simulink model "Receive1"  (R2021a)
settings: Solver=VariableStepAuto  StartTime=0.0  StopTime=20000  RelTol=1e-3
values from neighbouring files (symbols this model uses):
  n_overlapped_channel = 2 * 1024    (= 2048)    [receive1_script.m]
  parallel_factor = 4    [receive1_script.m]
libraries: xbsIndex_r4 x522, xrbsSSR_Library x15, dspsrcs4 x12
(part 2 of 4)

== system Receive1/beat_dphi2 ==
  w_addr : Inport
  w_data : Inport  Port=2
  we : Inport  Port=3
  tvalid_in : Inport  Port=4
  AddSub : xbsIndex_r4/AddSub  mode=Addition  use_carryin=off  use_carryout=off  en=off  latency=2  precision=User Defined  arith_type=Unsigned  n_bits=16  bin_pt=0  quantization=Truncate  overflow=Wrap  use_behavioral_HDL=off  hw_selection=Fabric  pipelined=off  dbl_ovrd=off  block_type=addsub
  Constant3 : xbsIndex_r4/Constant  const=0  gui_display_data_type=Boolean  arith_type=Boolean  n_bits=16  bin_pt=14  preci_type=Single  exp_width=8  frac_width=24  explicit_period=on  period=1  equ=P=C  opselect=C  inp2=PCIN>>17  opr=+  inp1=P  carry=CIN  dbl_ovrd=off  block_type=constant
  Constant5 : xbsIndex_r4/Constant  const=0  gui_display_data_type=Fixed-point  arith_type=Unsigned  n_bits=16  bin_pt=0  preci_type=Single  exp_width=8  frac_width=24  explicit_period=on  period=1  equ=P=C  opselect=C  inp2=PCIN>>17  opr=+  inp1=P  carry=CIN  dbl_ovrd=off  block_type=constant
  Constant6 : xbsIndex_r4/Constant  const=1  gui_display_data_type=Boolean  arith_type=Boolean  n_bits=16  bin_pt=14  preci_type=Single  exp_width=8  frac_width=24  explicit_period=on  period=1  equ=P=C  opselect=C  inp2=PCIN>>17  opr=+  inp1=P  carry=CIN  dbl_ovrd=off  block_type=constant
  Constant8 : xbsIndex_r4/Constant  const=0  gui_display_data_type=Fixed-point  arith_type=Unsigned  n_bits=16  bin_pt=0  preci_type=Single  exp_width=8  frac_width=24  explicit_period=on  period=1  equ=P=C  opselect=C  inp2=PCIN>>17  opr=+  inp1=P  carry=CIN  dbl_ovrd=off  block_type=constant
  Convert2 : xbsIndex_r4/Convert  gui_display_data_type=Fixed-point  arith_type="Signed  (2's comp)"  n_bits=18  bin_pt=15  float_type=Single  exp_bits=8  fraction_bits=24  quantization=Truncate  overflow=Wrap  en=off  latency=0  pipeline=off  dbl_ovrd=off  block_type=convert
  Counter2 : xbsIndex_r4/Counter  cnt_type=Free Running  cnt_to=Inf  operation=Up  start_count=0  cnt_by_val=1  arith_type=Unsigned  n_bits=9  bin_pt=0  load_pin=off  rst=on  en=on  explicit_period=on  period=1  use_behavioral_HDL=off  implementation=Fabric  dbl_ovrd=off  block_type=counter
  Delay{1,16,37..38} (4 alike) : xbsIndex_r4/Delay  rst=off  infoeditControl=Selection of Reset will increase slice count due to use of real FFs and instead of SRLs  en=off  latency=1  reg_retiming=off  dbl_ovrd=off  block_type=delay
  Delay17 : xbsIndex_r4/Delay  rst=off  infoeditControl=Selection of Reset will increase slice count due to use of real FFs and instead of SRLs  en=off  latency=n_overlapped_channel/parallel_factor-2-1-1  reg_retiming=off  dbl_ovrd=off  block_type=delay
  Dual Port RAM : xbsIndex_r4/Dual Port RAM  depth=n_overlapped_channel/parallel_factor  initVector=beat_dphi_uint16_2  distributed_mem=Block RAM  init_a=0  init_b=0  rst_a=off  rst_b=off  en_a=off  en_b=off  latency=1  write_mode_A=Read Before Write  write_mode_B=Read Before Write  optimize=Area  dbl_ovrd=off  simulation_type=fast_sim  block_type=dpram
  FIFO4 : xbsIndex_r4/FIFO  mem_type=Block RAM  performance_options=Standard_FIFO  embedded_registers=off  depth=1K  percent_nbits=1  rst=off  rst_latency=2  en=off  use_dcount=off  use_percent_full_port=off  use_almost_empty=off  almost_empty_thresh=2  use_almost_full=off  use_rd_rst_busy=off  use_wr_rst_busy=off  almost_full_thresh=14  explicit_period=off  dbl_ovrd=off  simulation_type=fast_sim  block_type=fifo
  Mux1 : xbsIndex_r4/Mux  inputs=2  en=off  latency=1  precision=User Defined  arith_type=Unsigned  n_bits=16  bin_pt=0  quantization=Truncate  overflow=Flag as error  dbl_ovrd=off  block_type=mux
  Mux2 : xbsIndex_r4/Mux  inputs=2  en=off  latency=1  precision=User Defined  arith_type=Unsigned  n_bits=16  bin_pt=0  quantization=Truncate  overflow=Flag as error  dbl_ovrd=off  block_type=mux
  Reinterpret2 : xbsIndex_r4/Reinterpret  force_arith_type=on  arith_type="Signed  (2's comp)"  force_bin_pt=on  bin_pt=15  block_type=reinterpret
  Terminator : Terminator
  Terminator11 : Terminator
  Terminator9 : Terminator
  rst_det : Subsystem
  beat_dphi : Outport
  wires:
  FIFO4/1 -> Mux1/3
  Reinterpret2/1 -> Convert2/1
  Delay17/1 -> FIFO4/3
  Delay38/1 -> Dual Port RAM/4
  Delay37/1 -> Dual Port RAM/5
  Delay16/1 -> Dual Port RAM/6
  Constant3/1 -> Dual Port RAM/3
  AddSub/1 -> FIFO4/1
  Constant6/1 -> FIFO4/2, Delay17/1
  FIFO4/3 -> Terminator11/1
  Constant8/1 -> Dual Port RAM/2
  FIFO4/2 -> Terminator9/1
  Dual Port RAM/2 -> Terminator/1
  Counter2/1 -> Dual Port RAM/1
  Constant5/1 -> Mux2/2, Mux1/2
  Mux2/1 -> AddSub/1
  w_data/1 -> Delay37/1
  Dual Port RAM/1 -> Mux2/3
  Convert2/1 -> beat_dphi/1
  w_addr/1 -> Delay38/1
  we/1 -> Delay16/1
  tvalid_in/1 -> rst_det/1(in), Delay1/1, Counter2/2
  rst_det/1(out) -> Counter2/1
  Delay1/1 -> Mux1/1, Mux2/1
  Mux1/1 -> Reinterpret2/1, AddSub/2

== system Receive1/beat_dphi3 ==
  w_addr : Inport
  w_data : Inport  Port=2
  we : Inport  Port=3
  tvalid_in : Inport  Port=4
  AddSub : xbsIndex_r4/AddSub  mode=Addition  use_carryin=off  use_carryout=off  en=off  latency=2  precision=User Defined  arith_type=Unsigned  n_bits=16  bin_pt=0  quantization=Truncate  overflow=Wrap  use_behavioral_HDL=off  hw_selection=Fabric  pipelined=off  dbl_ovrd=off  block_type=addsub
  Constant3 : xbsIndex_r4/Constant  const=0  gui_display_data_type=Boolean  arith_type=Boolean  n_bits=16  bin_pt=14  preci_type=Single  exp_width=8  frac_width=24  explicit_period=on  period=1  equ=P=C  opselect=C  inp2=PCIN>>17  opr=+  inp1=P  carry=CIN  dbl_ovrd=off  block_type=constant
  Constant5 : xbsIndex_r4/Constant  const=0  gui_display_data_type=Fixed-point  arith_type=Unsigned  n_bits=16  bin_pt=0  preci_type=Single  exp_width=8  frac_width=24  explicit_period=on  period=1  equ=P=C  opselect=C  inp2=PCIN>>17  opr=+  inp1=P  carry=CIN  dbl_ovrd=off  block_type=constant
  Constant6 : xbsIndex_r4/Constant  const=1  gui_display_data_type=Boolean  arith_type=Boolean  n_bits=16  bin_pt=14  preci_type=Single  exp_width=8  frac_width=24  explicit_period=on  period=1  equ=P=C  opselect=C  inp2=PCIN>>17  opr=+  inp1=P  carry=CIN  dbl_ovrd=off  block_type=constant
  Constant8 : xbsIndex_r4/Constant  const=0  gui_display_data_type=Fixed-point  arith_type=Unsigned  n_bits=16  bin_pt=0  preci_type=Single  exp_width=8  frac_width=24  explicit_period=on  period=1  equ=P=C  opselect=C  inp2=PCIN>>17  opr=+  inp1=P  carry=CIN  dbl_ovrd=off  block_type=constant
  Convert2 : xbsIndex_r4/Convert  gui_display_data_type=Fixed-point  arith_type="Signed  (2's comp)"  n_bits=18  bin_pt=15  float_type=Single  exp_bits=8  fraction_bits=24  quantization=Truncate  overflow=Wrap  en=off  latency=0  pipeline=off  dbl_ovrd=off  block_type=convert
  Counter2 : xbsIndex_r4/Counter  cnt_type=Free Running  cnt_to=Inf  operation=Up  start_count=0  cnt_by_val=1  arith_type=Unsigned  n_bits=9  bin_pt=0  load_pin=off  rst=on  en=on  explicit_period=on  period=1  use_behavioral_HDL=off  implementation=Fabric  dbl_ovrd=off  block_type=counter
  Delay{1,16,37..38} (4 alike) : xbsIndex_r4/Delay  rst=off  infoeditControl=Selection of Reset will increase slice count due to use of real FFs and instead of SRLs  en=off  latency=1  reg_retiming=off  dbl_ovrd=off  block_type=delay
  Delay17 : xbsIndex_r4/Delay  rst=off  infoeditControl=Selection of Reset will increase slice count due to use of real FFs and instead of SRLs  en=off  latency=n_overlapped_channel/parallel_factor-2-1-1  reg_retiming=off  dbl_ovrd=off  block_type=delay
  Dual Port RAM : xbsIndex_r4/Dual Port RAM  depth=n_overlapped_channel/parallel_factor  initVector=beat_dphi_uint16_3  distributed_mem=Block RAM  init_a=0  init_b=0  rst_a=off  rst_b=off  en_a=off  en_b=off  latency=1  write_mode_A=Read Before Write  write_mode_B=Read Before Write  optimize=Area  dbl_ovrd=off  simulation_type=fast_sim  block_type=dpram
  FIFO4 : xbsIndex_r4/FIFO  mem_type=Block RAM  performance_options=Standard_FIFO  embedded_registers=off  depth=1K  percent_nbits=1  rst=off  rst_latency=2  en=off  use_dcount=off  use_percent_full_port=off  use_almost_empty=off  almost_empty_thresh=2  use_almost_full=off  use_rd_rst_busy=off  use_wr_rst_busy=off  almost_full_thresh=14  explicit_period=off  dbl_ovrd=off  simulation_type=fast_sim  block_type=fifo
  Mux1 : xbsIndex_r4/Mux  inputs=2  en=off  latency=1  precision=User Defined  arith_type=Unsigned  n_bits=16  bin_pt=0  quantization=Truncate  overflow=Flag as error  dbl_ovrd=off  block_type=mux
  Mux2 : xbsIndex_r4/Mux  inputs=2  en=off  latency=1  precision=User Defined  arith_type=Unsigned  n_bits=16  bin_pt=0  quantization=Truncate  overflow=Flag as error  dbl_ovrd=off  block_type=mux
  Reinterpret2 : xbsIndex_r4/Reinterpret  force_arith_type=on  arith_type="Signed  (2's comp)"  force_bin_pt=on  bin_pt=15  block_type=reinterpret
  Terminator : Terminator
  Terminator11 : Terminator
  Terminator9 : Terminator
  rst_det : Subsystem
  beat_dphi : Outport
  wires:
  FIFO4/1 -> Mux1/3
  Reinterpret2/1 -> Convert2/1
  Delay17/1 -> FIFO4/3
  Delay38/1 -> Dual Port RAM/4
  Delay37/1 -> Dual Port RAM/5
  Delay16/1 -> Dual Port RAM/6
  Constant3/1 -> Dual Port RAM/3
  AddSub/1 -> FIFO4/1
  Constant6/1 -> FIFO4/2, Delay17/1
  FIFO4/3 -> Terminator11/1
  Constant8/1 -> Dual Port RAM/2
  FIFO4/2 -> Terminator9/1
  Dual Port RAM/2 -> Terminator/1
  Counter2/1 -> Dual Port RAM/1
  Constant5/1 -> Mux2/2, Mux1/2
  Mux2/1 -> AddSub/1
  w_data/1 -> Delay37/1
  Dual Port RAM/1 -> Mux2/3
  Convert2/1 -> beat_dphi/1
  w_addr/1 -> Delay38/1
  we/1 -> Delay16/1
  tvalid_in/1 -> rst_det/1(in), Delay1/1, Counter2/2
  rst_det/1(out) -> Counter2/1
  Delay1/1 -> Mux1/1, Mux2/1
  Mux1/1 -> Reinterpret2/1, AddSub/2

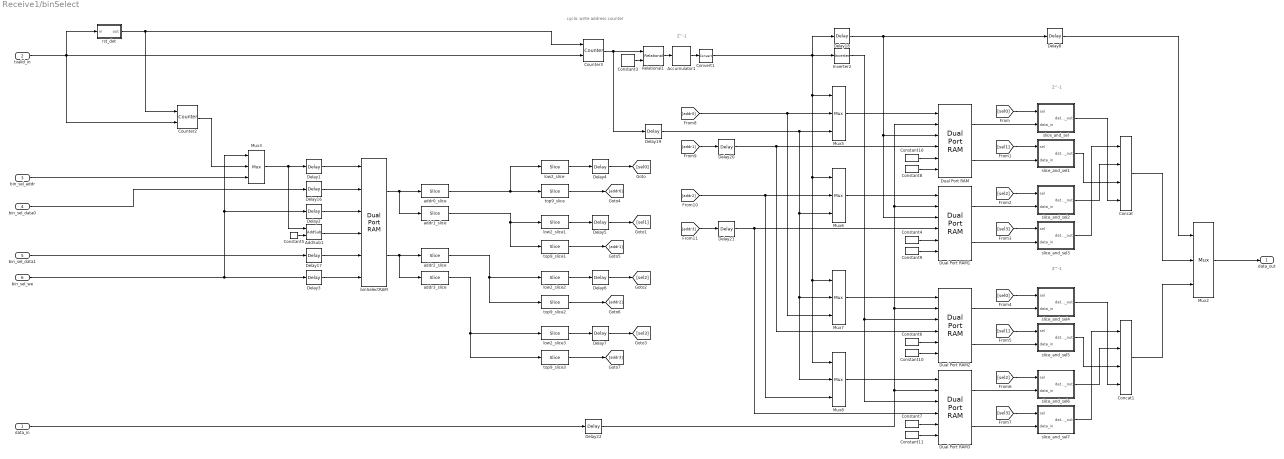
== system Receive1/binSelect ==
  note: Z^-1
  note: Z^-1
  note: Z^-1
  note: cyclic write address counter
  data_in : Inport
  tvalid_in : Inport  Port=2
  bin_sel_addr : Inport  Port=3
  bin_sel_data0 : Inport  Port=4
  bin_sel_data1 : Inport  Port=5
  bin_sel_we : Inport  Port=6
  Accumulator1 : xbsIndex_r4/Accumulator  operation=Add  n_bits=1  overflow=Wrap  scale=1  rst=off  hasbypass=off  infoeditControl=reset for floating point data type must be asserted for a minimum of 2 cycles  en=off  latency=1  msb_inp=100  msb=100  lsb=-100  use_behavioral_HDL=on  implementation=Fabric  dbl_ovrd=off  block_type=accum
  AddSub1 : xbsIndex_r4/AddSub  mode=Addition  use_carryin=off  use_carryout=off  en=off  latency=1  precision=User Defined  arith_type=Unsigned  n_bits=10  bin_pt=0  quantization=Truncate  overflow=Wrap  use_behavioral_HDL=on  hw_selection=Fabric  pipelined=on  dbl_ovrd=off  block_type=addsub
      settings: SourceProductName=Attempt to write the readonly database /home/ugrad/.matlab/R2018a/slblocks_master.db. (attempt to write a readonly database)
  Concat : xbsIndex_r4/Concat  num_inputs=4  dbl_ovrd=off  block_type=concat
  Concat1 : xbsIndex_r4/Concat  num_inputs=4  dbl_ovrd=off  block_type=concat
  Constant{8..11} (4 alike) : xbsIndex_r4/Constant  const=0  gui_display_data_type=Boolean  arith_type=Boolean  n_bits=1  bin_pt=0  preci_type=Single  exp_width=8  frac_width=24  explicit_period=on  period=1  equ=P=C  opselect=C  inp2=PCIN>>17  opr=+  inp1=P  carry=CIN  dbl_ovrd=off  block_type=constant
      settings: SourceProductName=Attempt to write the readonly database /home/ugrad/.matlab/R2018a/slblocks_master.db. (attempt to write a readonly database)
  Constant{4,6..7,16} (4 alike) : xbsIndex_r4/Constant  const=0  gui_display_data_type=Fixed-point  arith_type=Unsigned  n_bits=216  bin_pt=0  preci_type=Single  exp_width=8  frac_width=24  explicit_period=on  period=1  equ=P=C  opselect=C  inp2=PCIN>>17  opr=+  inp1=P  carry=CIN  dbl_ovrd=off  block_type=constant
      settings: SourceProductName=Attempt to write the readonly database /home/ugrad/.matlab/R2018a/slblocks_master.db. (attempt to write a readonly database)
  Constant3 : xbsIndex_r4/Constant  const=n_overlapped_channel/parallel_factor - 1  gui_display_data_type=Fixed-point  arith_type=Unsigned  n_bits=9  bin_pt=0  preci_type=Single  exp_width=8  frac_width=24  explicit_period=on  period=1  equ=P=C  opselect=C  inp2=PCIN>>17  opr=+  inp1=P  carry=CIN  dbl_ovrd=off  block_type=constant
  Constant5 : xbsIndex_r4/Constant  const=1  gui_display_data_type=Fixed-point  arith_type=Unsigned  n_bits=10  bin_pt=0  preci_type=Single  exp_width=8  frac_width=24  explicit_period=on  period=1  equ=P=C  opselect=C  inp2=PCIN>>17  opr=+  inp1=P  carry=CIN  dbl_ovrd=off  block_type=constant
      settings: SourceProductName=Attempt to write the readonly database /home/ugrad/.matlab/R2018a/slblocks_master.db. (attempt to write a readonly database)
  Convert1 : xbsIndex_r4/Convert  gui_display_data_type=Boolean  arith_type=Boolean  n_bits=16  bin_pt=14  float_type=Single  exp_bits=8  fraction_bits=24  quantization=Truncate  overflow=Wrap  en=off  latency=1  pipeline=off  dbl_ovrd=off  block_type=convert
  Counter2 : xbsIndex_r4/Counter  cnt_type=Free Running  cnt_to=Inf  operation=Up  start_count=0  cnt_by_val=2  arith_type=Unsigned  n_bits=10  bin_pt=0  load_pin=off  rst=on  en=on  explicit_period=on  period=1  use_behavioral_HDL=off  implementation=Fabric  dbl_ovrd=off  block_type=counter
  Counter3 : xbsIndex_r4/Counter  cnt_type=Free Running  cnt_to=Inf  operation=Up  start_count=0  cnt_by_val=1  arith_type=Unsigned  n_bits=9  bin_pt=0  load_pin=off  rst=on  en=on  explicit_period=on  period=1  use_behavioral_HDL=off  implementation=Fabric  dbl_ovrd=off  block_type=counter
  Delay{1,18,20..21} (4 alike) : xbsIndex_r4/Delay  rst=off  infoeditControl=Selection of Reset will increase slice count due to use of real FFs and instead of SRLs  en=off  latency=1  reg_retiming=off  dbl_ovrd=off  block_type=delay
  Delay{2..8,16..17} (9 alike) : xbsIndex_r4/Delay  rst=off  infoeditControl=Selection of Reset will increase slice count due to use of real FFs and instead of SRLs  en=off  latency=2  reg_retiming=off  dbl_ovrd=off  block_type=delay
  Delay19 : xbsIndex_r4/Delay  rst=off  infoeditControl=Selection of Reset will increase slice count due to use of real FFs and instead of SRLs  en=off  latency=3  reg_retiming=off  dbl_ovrd=off  block_type=delay
  Delay22 : xbsIndex_r4/Delay  rst=off  infoeditControl=Selection of Reset will increase slice count due to use of real FFs and instead of SRLs  en=off  latency=4  reg_retiming=off  dbl_ovrd=off  block_type=delay
  Dual Port RAM{,1..3} (4 alike) : xbsIndex_r4/Dual Port RAM  depth=n_overlapped_channel/parallel_factor  initVector=0  distributed_mem=Block RAM  init_a=0  init_b=0  rst_a=off  rst_b=off  en_a=off  en_b=off  latency=1  write_mode_A=Read Before Write  write_mode_B=Read Before Write  optimize=Area  dbl_ovrd=off  simulation_type=fast_sim  block_type=dpram
  Inverter2 : xbsIndex_r4/Inverter  en=off  latency=1  dbl_ovrd=off  block_type=inv
  Mux{2..3,5..8} (6 alike) : xbsIndex_r4/Mux  inputs=2  en=off  latency=1  precision=Full  arith_type=Unsigned  n_bits=16  bin_pt=14  quantization=Truncate  overflow=Wrap  dbl_ovrd=off  block_type=mux
  Relational1 : xbsIndex_r4/Relational  mode=a=b  op_type=Ufix  en=off  latency=1  dbl_ovrd=off  block_type=relational
  addr0_slice : xbsIndex_r4/Slice  nbits=11  boolean_output=off  mode=Lower Bit Location + Width  bit1=0  base1=MSB of Input  bit0=0  base0=LSB of Input  dbl_ovrd=off  block_type=slice
  addr1_slice : xbsIndex_r4/Slice  nbits=11  boolean_output=off  mode=Lower Bit Location + Width  bit1=0  base1=MSB of Input  bit0=11  base0=LSB of Input  dbl_ovrd=off  block_type=slice
  addr2_slice : xbsIndex_r4/Slice  nbits=11  boolean_output=off  mode=Lower Bit Location + Width  bit1=0  base1=MSB of Input  bit0=0  base0=LSB of Input  dbl_ovrd=off  block_type=slice
  addr3_slice : xbsIndex_r4/Slice  nbits=11  boolean_output=off  mode=Lower Bit Location + Width  bit1=0  base1=MSB of Input  bit0=11  base0=LSB of Input  dbl_ovrd=off  block_type=slice
  binSelectRAM : xbsIndex_r4/Dual Port RAM  depth=2*n_overlapped_channel/parallel_factor  initVector=bin_map  distributed_mem=Block RAM  init_a=0  init_b=0  rst_a=off  rst_b=off  en_a=off  en_b=off  latency=1  write_mode_A=Read Before Write  write_mode_B=Read Before Write  optimize=Area  dbl_ovrd=off  simulation_type=fast_sim  block_type=dpram
  low2_slice{,1..3} (4 alike) : xbsIndex_r4/Slice  nbits=2  boolean_output=off  mode=Lower Bit Location + Width  bit1=0  base1=MSB of Input  bit0=0  base0=LSB of Input  dbl_ovrd=off  block_type=slice
  rst_det : Subsystem
  slice_and_sel : Subsystem
  slice_and_sel1 : Subsystem
  slice_and_sel2 : Subsystem
  slice_and_sel3 : Subsystem
  slice_and_sel4 : Subsystem
  slice_and_sel5 : Subsystem
  slice_and_sel6 : Subsystem
  slice_and_sel7 : Subsystem
  top9_slice{,1..3} (4 alike) : xbsIndex_r4/Slice  nbits=9  boolean_output=off  mode=Lower Bit Location + Width  bit1=0  base1=MSB of Input  bit0=2  base0=LSB of Input  dbl_ovrd=off  block_type=slice
  data_out : Outport
  wires:
  [sel0] -> slice_and_sel/1(sel)
  Dual Port RAM/1 -> slice_and_sel/2(data_in)
  Dual Port RAM/2 -> slice_and_sel1/2(data_in)
  Dual Port RAM1/1 -> slice_and_sel2/2(data_in)
  Dual Port RAM1/2 -> slice_and_sel3/2(data_in)
  [sel1] -> slice_and_sel1/1(sel)
  [sel2] -> slice_and_sel2/1(sel)
  [sel3] -> slice_and_sel3/1(sel)
  slice_and_sel/1(data_out) -> Concat/4
  slice_and_sel1/1(data_out) -> Concat/3
  slice_and_sel2/1(data_out) -> Concat/2
  slice_and_sel3/1(data_out) -> Concat/1
  Dual Port RAM2/2 -> slice_and_sel5/2(data_in)
  slice_and_sel5/1(data_out) -> Concat1/3
  [sel0] -> slice_and_sel4/1(sel)
  Dual Port RAM2/1 -> slice_and_sel4/2(data_in)
  slice_and_sel7/1(data_out) -> Concat1/1
  [sel3] -> slice_and_sel7/1(sel)
  Dual Port RAM3/2 -> slice_and_sel7/2(data_in)
  [sel2] -> slice_and_sel6/1(sel)
  Dual Port RAM3/1 -> slice_and_sel6/2(data_in)
  [sel1] -> slice_and_sel5/1(sel)
  slice_and_sel4/1(data_out) -> Concat1/4
  slice_and_sel6/1(data_out) -> Concat1/2
  Concat/1 -> Mux2/2
  Concat1/1 -> Mux2/3
  Mux2/1 -> data_out/1
  Constant5/1 -> AddSub1/2
  AddSub1/1 -> binSelectRAM/4
  Delay1/1 -> binSelectRAM/1
  Mux3/1 -> Delay1/1, AddSub1/1
  Counter2/1 -> Mux3/2
  bin_sel_we/1 -> Delay2/1, Mux3/1, Delay3/1
  bin_sel_addr/1 -> Mux3/3
  Delay3/1 -> binSelectRAM/6
  Delay2/1 -> binSelectRAM/3
  Delay16/1 -> binSelectRAM/2
  Delay17/1 -> binSelectRAM/5
  bin_sel_data0/1 -> Delay16/1
  bin_sel_data1/1 -> Delay17/1
  binSelectRAM/1 -> addr0_slice/1, addr1_slice/1
  binSelectRAM/2 -> addr2_slice/1, addr3_slice/1
  addr0_slice/1 -> top9_slice/1, low2_slice/1
  addr1_slice/1 -> top9_slice1/1, low2_slice1/1
  addr2_slice/1 -> top9_slice2/1, low2_slice2/1
  addr3_slice/1 -> top9_slice3/1, low2_slice3/1
  top9_slice3/1 -> [addr3]
  top9_slice/1 -> [addr0]
  top9_slice1/1 -> [addr1]
  top9_slice2/1 -> [addr2]
  Mux5/1 -> Dual Port RAM/1
  Mux6/1 -> Dual Port RAM1/1
  Mux7/1 -> Dual Port RAM2/1
  Mux8/1 -> Dual Port RAM3/1
  Constant3/1 -> Relational1/2
  Accumulator1/1 -> Convert1/1
  Counter3/1 -> Delay19/1, Relational1/1
  Relational1/1 -> Accumulator1/1
  Constant16/1 -> Dual Port RAM/5
  Constant4/1 -> Dual Port RAM1/5
  Constant6/1 -> Dual Port RAM2/5
  Constant7/1 -> Dual Port RAM3/5
  Constant8/1 -> Dual Port RAM/6
  Constant9/1 -> Dual Port RAM1/6
  Constant10/1 -> Dual Port RAM2/6
  Constant11/1 -> Dual Port RAM3/6
  Convert1/1 -> Mux5/1, Mux8/1, Mux7/1, Mux6/1, Delay18/1, Inverter2/1
  Delay19/1 -> Mux8/2, Mux7/2, Mux6/3, Mux5/3
  Inverter2/1 -> Dual Port RAM2/3, Dual Port RAM3/3
  Delay18/1 -> Dual Port RAM1/3, Dual Port RAM/3, Delay8/1
  [addr0] -> Mux5/2, Mux7/3
  [addr1] -> Delay20/1
  [addr2] -> Mux6/2, Mux8/3
  [addr3] -> Delay21/1
  Delay20/1 -> Dual Port RAM/4, Dual Port RAM2/4
  Delay21/1 -> Dual Port RAM1/4, Dual Port RAM3/4
  data_in/1 -> Delay22/1
  Delay22/1 -> Dual Port RAM/2, Dual Port RAM1/2, Dual Port RAM2/2, Dual Port RAM3/2
  tvalid_in/1 -> Counter3/2, Counter2/2, rst_det/1(in)
  rst_det/1(out) -> Counter2/1, Counter3/1
  low2_slice/1 -> Delay4/1
  Delay4/1 -> [sel0]
  Delay5/1 -> [sel1]
  low2_slice1/1 -> Delay5/1
  Delay6/1 -> [sel2]
  low2_slice2/1 -> Delay6/1
  Delay7/1 -> [sel3]
  low2_slice3/1 -> Delay7/1
  Delay8/1 -> Mux2/1

== system Receive1/delayCounter ==
  note: Counter that is enabled after the first rising edge1, and disabled after the first rising edge2. Need to calibrate the initial value of counter before getting desired delay value.
  edge1 : Inport
  edge2 : Inport  Port=2
  Counter1 : xbsIndex_r4/Counter  cnt_type=Free Running  cnt_to=Inf  operation=Up  start_count=0  cnt_by_val=1  arith_type=Unsigned  n_bits=12  bin_pt=0  load_pin=off  rst=off  en=on  explicit_period=on  period=1  use_behavioral_HDL=off  implementation=DSP48  dbl_ovrd=off  block_type=counter
  Logical : xbsIndex_r4/Logical  logical_function=XOR  inputs=2  en=off  latency=1  precision=User Defined  arith_type=Boolean  n_bits=1  bin_pt=0  align_bp=on  dbl_ovrd=off  block_type=logical
  Register1 : xbsIndex_r4/Register  init=0  rst=off  en=on  dbl_ovrd=off  block_type=register
  Register2 : xbsIndex_r4/Register  init=0  rst=off  en=on  dbl_ovrd=off  block_type=register
  const1 : xbsIndex_r4/Constant  const=1  gui_display_data_type=Boolean  arith_type=Boolean  n_bits=18  bin_pt=16  preci_type=Single  exp_width=8  frac_width=24  explicit_period=on  period=1  equ=P=C  opselect=C  inp2=PCIN>>17  opr=+  inp1=P  carry=CIN  dbl_ovrd=off  block_type=constant
  delay : Outport
  wires:
  Counter1/1 -> delay/1
  Register2/1 -> Logical/2
  Logical/1 -> Counter1/1
  const1/1 -> Register1/1, Register2/1
  Register1/1 -> Logical/1
  edge2/1 -> Register2/2
  edge1/1 -> Register1/2

== system Receive1/delayCounter1 ==
  note: Counter that is enabled after the first rising edge1, and disabled after the first rising edge2. Need to calibrate the initial value of counter before getting desired delay value.
  edge1 : Inport
  edge2 : Inport  Port=2
  Counter1 : xbsIndex_r4/Counter  cnt_type=Free Running  cnt_to=Inf  operation=Up  start_count=0  cnt_by_val=1  arith_type=Unsigned  n_bits=12  bin_pt=0  load_pin=off  rst=off  en=on  explicit_period=on  period=1  use_behavioral_HDL=off  implementation=DSP48  dbl_ovrd=off  block_type=counter
  Logical : xbsIndex_r4/Logical  logical_function=XOR  inputs=2  en=off  latency=1  precision=User Defined  arith_type=Boolean  n_bits=1  bin_pt=0  align_bp=on  dbl_ovrd=off  block_type=logical
  Register1 : xbsIndex_r4/Register  init=0  rst=off  en=on  dbl_ovrd=off  block_type=register
  Register2 : xbsIndex_r4/Register  init=0  rst=off  en=on  dbl_ovrd=off  block_type=register
  const1 : xbsIndex_r4/Constant  const=1  gui_display_data_type=Boolean  arith_type=Boolean  n_bits=18  bin_pt=16  preci_type=Single  exp_width=8  frac_width=24  explicit_period=on  period=1  equ=P=C  opselect=C  inp2=PCIN>>17  opr=+  inp1=P  carry=CIN  dbl_ovrd=off  block_type=constant
  delay : Outport
  wires:
  Counter1/1 -> delay/1
  Register2/1 -> Logical/2
  Logical/1 -> Counter1/1
  const1/1 -> Register1/1, Register2/1
  Register1/1 -> Logical/1
  edge2/1 -> Register2/2
  edge1/1 -> Register1/2

== system Receive1/rst_det ==
  in : Inport
  Inverter : xbsIndex_r4/Inverter  en=off  latency=1  dbl_ovrd=off  block_type=inv
  Logical : xbsIndex_r4/Logical  logical_function=AND  inputs=2  en=off  latency=1  precision=User Defined  arith_type=Boolean  n_bits=1  bin_pt=0  align_bp=on  dbl_ovrd=off  block_type=logical
  Logical1 : xbsIndex_r4/Logical  logical_function=XOR  inputs=2  en=off  latency=1  precision=User Defined  arith_type=Boolean  n_bits=1  bin_pt=0  align_bp=on  dbl_ovrd=off  block_type=logical
  Register : xbsIndex_r4/Register  init=0  rst=off  en=off  dbl_ovrd=off  block_type=register
  out : Outport
  wires:
  Register/1 -> Logical1/2, Logical/2
  Inverter/1 -> Logical1/1, Register/1
  Logical1/1 -> Logical/1
  in/1 -> Inverter/1
  Logical/1 -> out/1

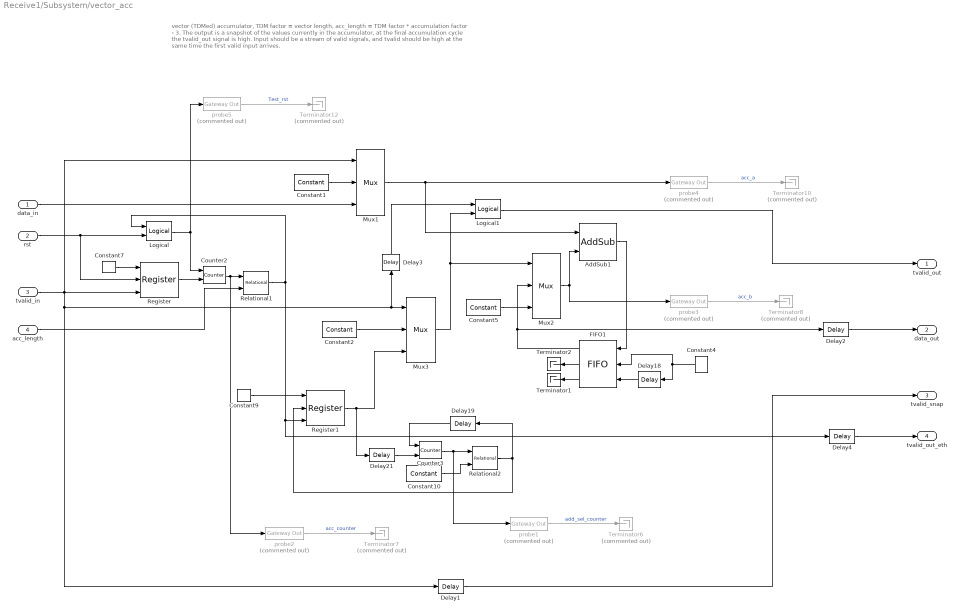
== system Receive1/Subsystem/vector_acc ==
  note: vector (TDMed) accumulator, TDM factor = vector length, acc_length = TDM factor * accumulation factor - 3.
      | The output is a snapshot of the values currently in the accumulator, at the final accumulation cycle the tvalid_out signal is high.
      | Input should be a stream of valid signals, and tvalid should be high at the same time the first valid input arrives.
  data_in : Inport
  rst : Inport  Port=2
  tvalid_in : Inport  Port=3
  acc_length : Inport  Port=4
  AddSub1 : xbsIndex_r4/AddSub  mode=Addition  use_carryin=off  use_carryout=off  en=off  latency=2  precision=User Defined  arith_type="Signed  (2's comp)"  n_bits=32  bin_pt=14  quantization=Truncate  overflow=Flag as error  use_behavioral_HDL=off  hw_selection=Fabric  pipelined=off  dbl_ovrd=off  block_type=addsub
  Constant1 : xbsIndex_r4/Constant  const=0  gui_display_data_type=Fixed-point  arith_type=Signed (2's comp)  n_bits=16  bin_pt=14  preci_type=Single  exp_width=8  frac_width=24  explicit_period=on  period=1  equ=P=C  opselect=C  inp2=PCIN>>17  opr=+  inp1=P  carry=CIN  dbl_ovrd=off  block_type=constant
  Constant10 : xbsIndex_r4/Constant  const=(n_overlapped_channel/parallel_factor-1)-2  gui_display_data_type=Fixed-point  arith_type=Unsigned  n_bits=16  bin_pt=0  preci_type=Single  exp_width=8  frac_width=24  explicit_period=on  period=1  equ=P=C  opselect=C  inp2=PCIN>>17  opr=+  inp1=P  carry=CIN  dbl_ovrd=off  block_type=constant
  Constant2 : xbsIndex_r4/Constant  const=1  gui_display_data_type=Boolean  arith_type=Boolean  n_bits=32  bin_pt=14  preci_type=Single  exp_width=8  frac_width=24  explicit_period=on  period=1  equ=P=C  opselect=C  inp2=PCIN>>17  opr=+  inp1=P  carry=CIN  dbl_ovrd=off  block_type=constant
  Constant4 : xbsIndex_r4/Constant  const=1  gui_display_data_type=Boolean  arith_type=Boolean  n_bits=16  bin_pt=14  preci_type=Single  exp_width=8  frac_width=24  explicit_period=on  period=1  equ=P=C  opselect=C  inp2=PCIN>>17  opr=+  inp1=P  carry=CIN  dbl_ovrd=off  block_type=constant
  Constant5 : xbsIndex_r4/Constant  const=0  gui_display_data_type=Fixed-point  arith_type=Signed (2's comp)  n_bits=32  bin_pt=14  preci_type=Single  exp_width=8  frac_width=24  explicit_period=on  period=1  equ=P=C  opselect=C  inp2=PCIN>>17  opr=+  inp1=P  carry=CIN  dbl_ovrd=off  block_type=constant
  Constant7 : xbsIndex_r4/Constant  const=1  gui_display_data_type=Boolean  arith_type=Boolean  n_bits=64  bin_pt=14  preci_type=Single  exp_width=8  frac_width=24  explicit_period=on  period=1  equ=P=C  opselect=C  inp2=PCIN>>17  opr=+  inp1=P  carry=CIN  dbl_ovrd=off  block_type=constant
  Constant9 : xbsIndex_r4/Constant  const=1  gui_display_data_type=Boolean  arith_type=Boolean  n_bits=64  bin_pt=14  preci_type=Single  exp_width=8  frac_width=24  explicit_period=on  period=1  equ=P=C  opselect=C  inp2=PCIN>>17  opr=+  inp1=P  carry=CIN  dbl_ovrd=off  block_type=constant
  Counter2 : xbsIndex_r4/Counter  cnt_type=Free Running  cnt_to=Inf  operation=Up  start_count=0  cnt_by_val=1  arith_type=Unsigned  n_bits=24  bin_pt=0  load_pin=off  rst=on  en=on  explicit_period=on  period=1  use_behavioral_HDL=off  implementation=Fabric  dbl_ovrd=off  block_type=counter
  Counter3 : xbsIndex_r4/Counter  cnt_type=Free Running  cnt_to=Inf  operation=Up  start_count=0  cnt_by_val=1  arith_type=Unsigned  n_bits=9  bin_pt=0  load_pin=off  rst=on  en=on  explicit_period=on  period=1  use_behavioral_HDL=off  implementation=Fabric  dbl_ovrd=off  block_type=counter
  Delay1 : xbsIndex_r4/Delay  rst=off  infoeditControl=Selection of Reset will increase slice count due to use of real FFs and instead of SRLs  en=off  latency=513  reg_retiming=off  dbl_ovrd=off  block_type=delay
  Delay18 : xbsIndex_r4/Delay  rst=off  infoeditControl=Selection of Reset will increase slice count due to use of real FFs and instead of SRLs  en=off  latency=n_overlapped_channel/parallel_factor-(2+1)-1  reg_retiming=off  dbl_ovrd=off  block_type=delay
  Delay19 : xbsIndex_r4/Delay  rst=off  infoeditControl=Selection of Reset will increase slice count due to use of real FFs and instead of SRLs  en=off  latency=2  reg_retiming=off  dbl_ovrd=off  block_type=delay
  Delay2 : xbsIndex_r4/Delay  rst=off  infoeditControl=Selection of Reset will increase slice count due to use of real FFs and instead of SRLs  en=off  latency=1  reg_retiming=off  dbl_ovrd=off  block_type=delay
  Delay21 : xbsIndex_r4/Delay  rst=off  infoeditControl=Selection of Reset will increase slice count due to use of real FFs and instead of SRLs  en=off  latency=1  reg_retiming=off  dbl_ovrd=off  block_type=delay
  Delay3 : xbsIndex_r4/Delay  rst=off  infoeditControl=Selection of Reset will increase slice count due to use of real FFs and instead of SRLs  en=off  latency=1  reg_retiming=off  dbl_ovrd=off  block_type=delay
  Delay4 : xbsIndex_r4/Delay  rst=off  infoeditControl=Selection of Reset will increase slice count due to use of real FFs and instead of SRLs  en=off  latency=2  reg_retiming=off  dbl_ovrd=off  block_type=delay
  FIFO1 : xbsIndex_r4/FIFO  mem_type=Block RAM  performance_options=Standard_FIFO  embedded_registers=off  depth=1K  percent_nbits=1  rst=off  rst_latency=2  en=off  use_dcount=off  use_percent_full_port=off  use_almost_empty=off  almost_empty_thresh=2  use_almost_full=off  use_rd_rst_busy=off  use_wr_rst_busy=off  almost_full_thresh=14  explicit_period=off  dbl_ovrd=off  simulation_type=fast_sim  block_type=fifo
  Logical : xbsIndex_r4/Logical  logical_function=OR  inputs=2  en=off  latency=2  precision=User Defined  arith_type=Boolean  n_bits=1  bin_pt=0  align_bp=on  dbl_ovrd=off  block_type=logical
  Logical1 : xbsIndex_r4/Logical  logical_function=AND  inputs=2  en=off  latency=1  precision=User Defined  arith_type=Boolean  n_bits=1  bin_pt=0  align_bp=on  dbl_ovrd=off  block_type=logical
  Mux1 : xbsIndex_r4/Mux  inputs=2  en=off  latency=1  precision=User Defined  arith_type="Signed  (2's comp)"  n_bits=16  bin_pt=14  quantization=Truncate  overflow=Flag as error  dbl_ovrd=off  block_type=mux
  Mux2 : xbsIndex_r4/Mux  inputs=2  en=off  latency=1  precision=User Defined  arith_type="Signed  (2's comp)"  n_bits=32  bin_pt=14  quantization=Truncate  overflow=Flag as error  dbl_ovrd=off  block_type=mux
  Mux3 : xbsIndex_r4/Mux  inputs=2  en=off  latency=1  precision=Full  arith_type=Unsigned  n_bits=1  bin_pt=0  quantization=Truncate  overflow=Wrap  dbl_ovrd=off  block_type=mux
  Register : xbsIndex_r4/Register  init=0  rst=on  en=on  dbl_ovrd=off  block_type=register
  Register1 : xbsIndex_r4/Register  init=0  rst=on  en=on  dbl_ovrd=off  block_type=register
  Relational1 : xbsIndex_r4/Relational  mode=a=b  op_type=Bool  en=off  latency=1  dbl_ovrd=off  block_type=relational
  Relational2 : xbsIndex_r4/Relational  mode=a=b  op_type=Bool  en=off  latency=1  dbl_ovrd=off  block_type=relational
  Terminator1 : Terminator
  Terminator{6..8,10,12} (5 alike) : Terminator  Commented=on
  Terminator2 : Terminator
  probe{1..5} (5 alike) : xbsIndex_r4/Gateway Out  Commented=on  inherit_from_input=off  hdl_port=on  rows=1  columns=1  UseAsDAC=off  DACChannel='1'  interface=None  automatic_assignment=on  address_offset=hex2dec('00')  intf_name=''  intf_description=''  timing_constraint=None  locs_specified=off  LOCs={}  io_standard={}  block_type=gatewayout
  tvalid_out : Outport
  data_out : Outport  Port=2
  tvalid_snap : Outport  Port=3
  tvalid_out_eth : Outport  Port=4
  wires:
  Register/1 -> Counter2/2
  Mux2/1 -> AddSub1/2, probe3/1
  Mux1/1 -> AddSub1/1, probe4/1
  Counter2/1 -> probe2/1, Relational1/1
  Constant5/1 -> Mux2/3
  FIFO1/3 -> Terminator1/1
  Constant7/1 -> Register/1
  FIFO1/2 -> Terminator2/1
  probe1/1 -> Terminator6/1  "add_sel_counter"
  probe2/1 -> Terminator7/1  "acc_counter"
  probe5/1 -> Terminator12/1  "Test_rst"
  Constant4/1 -> Delay18/1, FIFO1/2
  Delay19/1 -> Counter3/1
  Delay21/1 -> Counter3/2
  Constant9/1 -> Register1/1
  Relational1/1 -> Logical/1, Delay4/1, Register1/3
  Counter3/1 -> probe1/1, Relational2/1
  Register1/1 -> Mux3/3, Delay21/1
  Delay18/1 -> FIFO1/3
  AddSub1/1 -> FIFO1/1
  Constant10/1 -> Relational2/2
  Relational2/1 -> Register1/2, Delay19/1
  rst/1 -> Logical/2, Register/2
  Logical/1 -> Counter2/1, probe5/1
  FIFO1/1 -> Mux2/2, Delay2/1
  probe4/1 -> Terminator10/1  "acc_a"
  data_in/1 -> Mux1/3
  probe3/1 -> Terminator8/1  "acc_b"
  acc_length/1 -> Relational1/2
  tvalid_in/1 -> Mux3/1, Delay3/1, Delay1/1, Register/3, Mux1/1
  Constant1/1 -> Mux1/2
  Delay1/1 -> tvalid_snap/1
  Mux3/1 -> Mux2/1, Logical1/2
  Constant2/1 -> Mux3/2
  Logical1/1 -> tvalid_out/1
  Delay2/1 -> data_out/1
  Delay3/1 -> Logical1/1
  Delay4/1 -> tvalid_out_eth/1

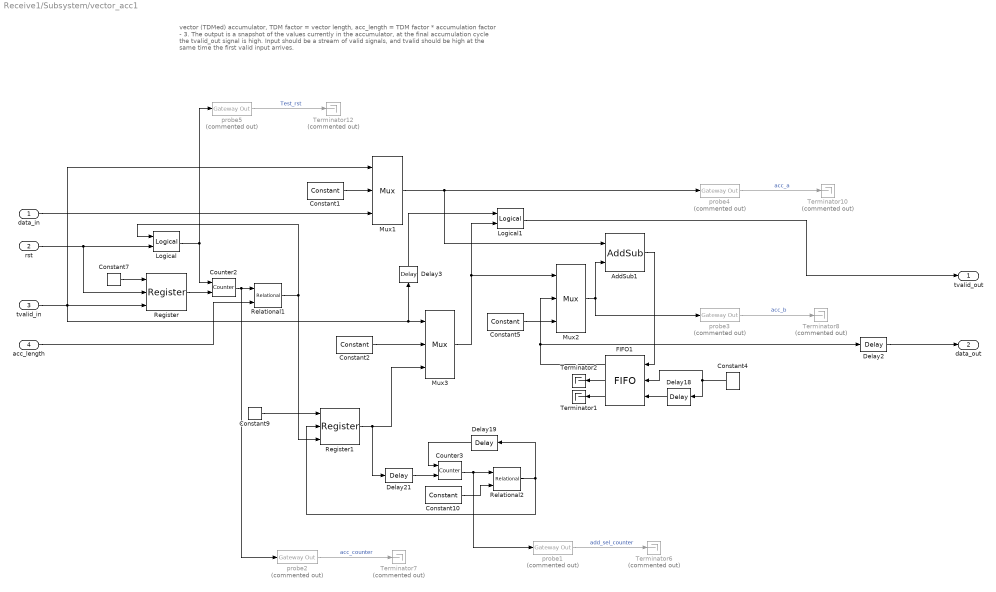
== system Receive1/Subsystem/vector_acc1 ==
  note: vector (TDMed) accumulator, TDM factor = vector length, acc_length = TDM factor * accumulation factor - 3.
      | The output is a snapshot of the values currently in the accumulator, at the final accumulation cycle the tvalid_out signal is high.
      | Input should be a stream of valid signals, and tvalid should be high at the same time the first valid input arrives.
  data_in : Inport
  rst : Inport  Port=2
  tvalid_in : Inport  Port=3
  acc_length : Inport  Port=4
  AddSub1 : xbsIndex_r4/AddSub  mode=Addition  use_carryin=off  use_carryout=off  en=off  latency=2  precision=User Defined  arith_type="Signed  (2's comp)"  n_bits=32  bin_pt=14  quantization=Truncate  overflow=Flag as error  use_behavioral_HDL=off  hw_selection=Fabric  pipelined=off  dbl_ovrd=off  block_type=addsub
  Constant1 : xbsIndex_r4/Constant  const=0  gui_display_data_type=Fixed-point  arith_type=Signed (2's comp)  n_bits=16  bin_pt=14  preci_type=Single  exp_width=8  frac_width=24  explicit_period=on  period=1  equ=P=C  opselect=C  inp2=PCIN>>17  opr=+  inp1=P  carry=CIN  dbl_ovrd=off  block_type=constant
  Constant10 : xbsIndex_r4/Constant  const=(n_overlapped_channel/parallel_factor-1)-2  gui_display_data_type=Fixed-point  arith_type=Unsigned  n_bits=16  bin_pt=0  preci_type=Single  exp_width=8  frac_width=24  explicit_period=on  period=1  equ=P=C  opselect=C  inp2=PCIN>>17  opr=+  inp1=P  carry=CIN  dbl_ovrd=off  block_type=constant
  Constant2 : xbsIndex_r4/Constant  const=1  gui_display_data_type=Boolean  arith_type=Boolean  n_bits=32  bin_pt=14  preci_type=Single  exp_width=8  frac_width=24  explicit_period=on  period=1  equ=P=C  opselect=C  inp2=PCIN>>17  opr=+  inp1=P  carry=CIN  dbl_ovrd=off  block_type=constant
  Constant4 : xbsIndex_r4/Constant  const=1  gui_display_data_type=Boolean  arith_type=Boolean  n_bits=16  bin_pt=14  preci_type=Single  exp_width=8  frac_width=24  explicit_period=on  period=1  equ=P=C  opselect=C  inp2=PCIN>>17  opr=+  inp1=P  carry=CIN  dbl_ovrd=off  block_type=constant
  Constant5 : xbsIndex_r4/Constant  const=0  gui_display_data_type=Fixed-point  arith_type=Signed (2's comp)  n_bits=32  bin_pt=14  preci_type=Single  exp_width=8  frac_width=24  explicit_period=on  period=1  equ=P=C  opselect=C  inp2=PCIN>>17  opr=+  inp1=P  carry=CIN  dbl_ovrd=off  block_type=constant
  Constant7 : xbsIndex_r4/Constant  const=1  gui_display_data_type=Boolean  arith_type=Boolean  n_bits=64  bin_pt=14  preci_type=Single  exp_width=8  frac_width=24  explicit_period=on  period=1  equ=P=C  opselect=C  inp2=PCIN>>17  opr=+  inp1=P  carry=CIN  dbl_ovrd=off  block_type=constant
  Constant9 : xbsIndex_r4/Constant  const=1  gui_display_data_type=Boolean  arith_type=Boolean  n_bits=64  bin_pt=14  preci_type=Single  exp_width=8  frac_width=24  explicit_period=on  period=1  equ=P=C  opselect=C  inp2=PCIN>>17  opr=+  inp1=P  carry=CIN  dbl_ovrd=off  block_type=constant
  Counter2 : xbsIndex_r4/Counter  cnt_type=Free Running  cnt_to=Inf  operation=Up  start_count=0  cnt_by_val=1  arith_type=Unsigned  n_bits=24  bin_pt=0  load_pin=off  rst=on  en=on  explicit_period=on  period=1  use_behavioral_HDL=off  implementation=Fabric  dbl_ovrd=off  block_type=counter
  Counter3 : xbsIndex_r4/Counter  cnt_type=Free Running  cnt_to=Inf  operation=Up  start_count=0  cnt_by_val=1  arith_type=Unsigned  n_bits=9  bin_pt=0  load_pin=off  rst=on  en=on  explicit_period=on  period=1  use_behavioral_HDL=off  implementation=Fabric  dbl_ovrd=off  block_type=counter
  Delay18 : xbsIndex_r4/Delay  rst=off  infoeditControl=Selection of Reset will increase slice count due to use of real FFs and instead of SRLs  en=off  latency=n_overlapped_channel/parallel_factor-(2+1)-1  reg_retiming=off  dbl_ovrd=off  block_type=delay
  Delay19 : xbsIndex_r4/Delay  rst=off  infoeditControl=Selection of Reset will increase slice count due to use of real FFs and instead of SRLs  en=off  latency=2  reg_retiming=off  dbl_ovrd=off  block_type=delay
  Delay2 : xbsIndex_r4/Delay  rst=off  infoeditControl=Selection of Reset will increase slice count due to use of real FFs and instead of SRLs  en=off  latency=1  reg_retiming=off  dbl_ovrd=off  block_type=delay
  Delay21 : xbsIndex_r4/Delay  rst=off  infoeditControl=Selection of Reset will increase slice count due to use of real FFs and instead of SRLs  en=off  latency=1  reg_retiming=off  dbl_ovrd=off  block_type=delay
  Delay3 : xbsIndex_r4/Delay  rst=off  infoeditControl=Selection of Reset will increase slice count due to use of real FFs and instead of SRLs  en=off  latency=1  reg_retiming=off  dbl_ovrd=off  block_type=delay
  FIFO1 : xbsIndex_r4/FIFO  mem_type=Block RAM  performance_options=Standard_FIFO  embedded_registers=off  depth=1K  percent_nbits=1  rst=off  rst_latency=2  en=off  use_dcount=off  use_percent_full_port=off  use_almost_empty=off  almost_empty_thresh=2  use_almost_full=off  use_rd_rst_busy=off  use_wr_rst_busy=off  almost_full_thresh=14  explicit_period=off  dbl_ovrd=off  simulation_type=fast_sim  block_type=fifo
  Logical : xbsIndex_r4/Logical  logical_function=OR  inputs=2  en=off  latency=2  precision=User Defined  arith_type=Boolean  n_bits=1  bin_pt=0  align_bp=on  dbl_ovrd=off  block_type=logical
  Logical1 : xbsIndex_r4/Logical  logical_function=AND  inputs=2  en=off  latency=1  precision=User Defined  arith_type=Boolean  n_bits=1  bin_pt=0  align_bp=on  dbl_ovrd=off  block_type=logical
  Mux1 : xbsIndex_r4/Mux  inputs=2  en=off  latency=1  precision=User Defined  arith_type="Signed  (2's comp)"  n_bits=16  bin_pt=14  quantization=Truncate  overflow=Flag as error  dbl_ovrd=off  block_type=mux
  Mux2 : xbsIndex_r4/Mux  inputs=2  en=off  latency=1  precision=User Defined  arith_type="Signed  (2's comp)"  n_bits=32  bin_pt=14  quantization=Truncate  overflow=Flag as error  dbl_ovrd=off  block_type=mux
  Mux3 : xbsIndex_r4/Mux  inputs=2  en=off  latency=1  precision=Full  arith_type=Unsigned  n_bits=1  bin_pt=0  quantization=Truncate  overflow=Wrap  dbl_ovrd=off  block_type=mux
  Register : xbsIndex_r4/Register  init=0  rst=on  en=on  dbl_ovrd=off  block_type=register
  Register1 : xbsIndex_r4/Register  init=0  rst=on  en=on  dbl_ovrd=off  block_type=register
  Relational1 : xbsIndex_r4/Relational  mode=a=b  op_type=Bool  en=off  latency=1  dbl_ovrd=off  block_type=relational
  Relational2 : xbsIndex_r4/Relational  mode=a=b  op_type=Bool  en=off  latency=1  dbl_ovrd=off  block_type=relational
  Terminator1 : Terminator
  Terminator{6..8,10,12} (5 alike) : Terminator  Commented=on
  Terminator2 : Terminator
  probe{1..5} (5 alike) : xbsIndex_r4/Gateway Out  Commented=on  inherit_from_input=off  hdl_port=on  rows=1  columns=1  UseAsDAC=off  DACChannel='1'  interface=None  automatic_assignment=on  address_offset=hex2dec('00')  intf_name=''  intf_description=''  timing_constraint=None  locs_specified=off  LOCs={}  io_standard={}  block_type=gatewayout
  tvalid_out : Outport
  data_out : Outport  Port=2
  wires:
  Register/1 -> Counter2/2
  Mux2/1 -> AddSub1/2, probe3/1
  Mux1/1 -> AddSub1/1, probe4/1
  Counter2/1 -> probe2/1, Relational1/1
  Constant5/1 -> Mux2/3
  FIFO1/3 -> Terminator1/1
  Constant7/1 -> Register/1
  FIFO1/2 -> Terminator2/1
  probe1/1 -> Terminator6/1  "add_sel_counter"
  probe2/1 -> Terminator7/1  "acc_counter"
  probe5/1 -> Terminator12/1  "Test_rst"
  Constant4/1 -> Delay18/1, FIFO1/2
  Delay19/1 -> Counter3/1
  Delay21/1 -> Counter3/2
  Constant9/1 -> Register1/1
  Relational1/1 -> Logical/1, Register1/3
  Counter3/1 -> probe1/1, Relational2/1
  Register1/1 -> Mux3/3, Delay21/1
  Delay18/1 -> FIFO1/3
  AddSub1/1 -> FIFO1/1
  Constant10/1 -> Relational2/2
  Relational2/1 -> Register1/2, Delay19/1
  rst/1 -> Logical/2, Register/2
  Logical/1 -> Counter2/1, probe5/1
  FIFO1/1 -> Mux2/2, Delay2/1
  probe4/1 -> Terminator10/1  "acc_a"
  data_in/1 -> Mux1/3
  probe3/1 -> Terminator8/1  "acc_b"
  acc_length/1 -> Relational1/2
  tvalid_in/1 -> Mux3/1, Delay3/1, Register/3, Mux1/1
  Constant1/1 -> Mux1/2
  Mux3/1 -> Mux2/1, Logical1/2
  Constant2/1 -> Mux3/2
  Logical1/1 -> tvalid_out/1
  Delay2/1 -> data_out/1
  Delay3/1 -> Logical1/1

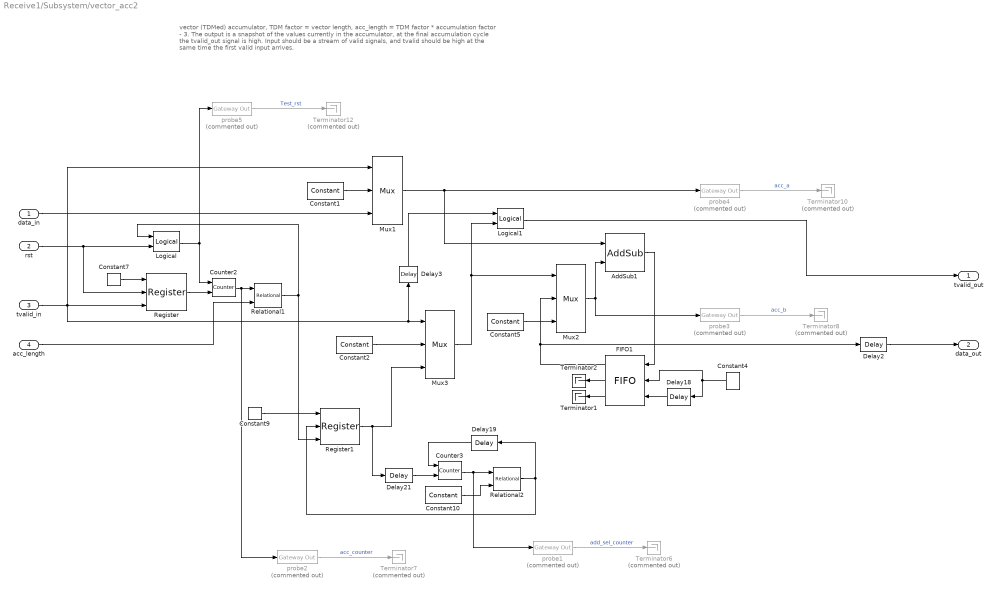
== system Receive1/Subsystem/vector_acc2 ==
  note: vector (TDMed) accumulator, TDM factor = vector length, acc_length = TDM factor * accumulation factor - 3.
      | The output is a snapshot of the values currently in the accumulator, at the final accumulation cycle the tvalid_out signal is high.
      | Input should be a stream of valid signals, and tvalid should be high at the same time the first valid input arrives.
  data_in : Inport
  rst : Inport  Port=2
  tvalid_in : Inport  Port=3
  acc_length : Inport  Port=4
  AddSub1 : xbsIndex_r4/AddSub  mode=Addition  use_carryin=off  use_carryout=off  en=off  latency=2  precision=User Defined  arith_type="Signed  (2's comp)"  n_bits=32  bin_pt=14  quantization=Truncate  overflow=Flag as error  use_behavioral_HDL=off  hw_selection=Fabric  pipelined=off  dbl_ovrd=off  block_type=addsub
  Constant1 : xbsIndex_r4/Constant  const=0  gui_display_data_type=Fixed-point  arith_type=Signed (2's comp)  n_bits=16  bin_pt=14  preci_type=Single  exp_width=8  frac_width=24  explicit_period=on  period=1  equ=P=C  opselect=C  inp2=PCIN>>17  opr=+  inp1=P  carry=CIN  dbl_ovrd=off  block_type=constant
  Constant10 : xbsIndex_r4/Constant  const=(n_overlapped_channel/parallel_factor-1)-2  gui_display_data_type=Fixed-point  arith_type=Unsigned  n_bits=16  bin_pt=0  preci_type=Single  exp_width=8  frac_width=24  explicit_period=on  period=1  equ=P=C  opselect=C  inp2=PCIN>>17  opr=+  inp1=P  carry=CIN  dbl_ovrd=off  block_type=constant
  Constant2 : xbsIndex_r4/Constant  const=1  gui_display_data_type=Boolean  arith_type=Boolean  n_bits=32  bin_pt=14  preci_type=Single  exp_width=8  frac_width=24  explicit_period=on  period=1  equ=P=C  opselect=C  inp2=PCIN>>17  opr=+  inp1=P  carry=CIN  dbl_ovrd=off  block_type=constant
  Constant4 : xbsIndex_r4/Constant  const=1  gui_display_data_type=Boolean  arith_type=Boolean  n_bits=16  bin_pt=14  preci_type=Single  exp_width=8  frac_width=24  explicit_period=on  period=1  equ=P=C  opselect=C  inp2=PCIN>>17  opr=+  inp1=P  carry=CIN  dbl_ovrd=off  block_type=constant
  Constant5 : xbsIndex_r4/Constant  const=0  gui_display_data_type=Fixed-point  arith_type=Signed (2's comp)  n_bits=32  bin_pt=14  preci_type=Single  exp_width=8  frac_width=24  explicit_period=on  period=1  equ=P=C  opselect=C  inp2=PCIN>>17  opr=+  inp1=P  carry=CIN  dbl_ovrd=off  block_type=constant
  Constant7 : xbsIndex_r4/Constant  const=1  gui_display_data_type=Boolean  arith_type=Boolean  n_bits=64  bin_pt=14  preci_type=Single  exp_width=8  frac_width=24  explicit_period=on  period=1  equ=P=C  opselect=C  inp2=PCIN>>17  opr=+  inp1=P  carry=CIN  dbl_ovrd=off  block_type=constant
  Constant9 : xbsIndex_r4/Constant  const=1  gui_display_data_type=Boolean  arith_type=Boolean  n_bits=64  bin_pt=14  preci_type=Single  exp_width=8  frac_width=24  explicit_period=on  period=1  equ=P=C  opselect=C  inp2=PCIN>>17  opr=+  inp1=P  carry=CIN  dbl_ovrd=off  block_type=constant
  Counter2 : xbsIndex_r4/Counter  cnt_type=Free Running  cnt_to=Inf  operation=Up  start_count=0  cnt_by_val=1  arith_type=Unsigned  n_bits=24  bin_pt=0  load_pin=off  rst=on  en=on  explicit_period=on  period=1  use_behavioral_HDL=off  implementation=Fabric  dbl_ovrd=off  block_type=counter
  Counter3 : xbsIndex_r4/Counter  cnt_type=Free Running  cnt_to=Inf  operation=Up  start_count=0  cnt_by_val=1  arith_type=Unsigned  n_bits=9  bin_pt=0  load_pin=off  rst=on  en=on  explicit_period=on  period=1  use_behavioral_HDL=off  implementation=Fabric  dbl_ovrd=off  block_type=counter
  Delay18 : xbsIndex_r4/Delay  rst=off  infoeditControl=Selection of Reset will increase slice count due to use of real FFs and instead of SRLs  en=off  latency=n_overlapped_channel/parallel_factor-(2+1)-1  reg_retiming=off  dbl_ovrd=off  block_type=delay
  Delay19 : xbsIndex_r4/Delay  rst=off  infoeditControl=Selection of Reset will increase slice count due to use of real FFs and instead of SRLs  en=off  latency=2  reg_retiming=off  dbl_ovrd=off  block_type=delay
  Delay2 : xbsIndex_r4/Delay  rst=off  infoeditControl=Selection of Reset will increase slice count due to use of real FFs and instead of SRLs  en=off  latency=1  reg_retiming=off  dbl_ovrd=off  block_type=delay
  Delay21 : xbsIndex_r4/Delay  rst=off  infoeditControl=Selection of Reset will increase slice count due to use of real FFs and instead of SRLs  en=off  latency=1  reg_retiming=off  dbl_ovrd=off  block_type=delay
  Delay3 : xbsIndex_r4/Delay  rst=off  infoeditControl=Selection of Reset will increase slice count due to use of real FFs and instead of SRLs  en=off  latency=1  reg_retiming=off  dbl_ovrd=off  block_type=delay
  FIFO1 : xbsIndex_r4/FIFO  mem_type=Block RAM  performance_options=Standard_FIFO  embedded_registers=off  depth=1K  percent_nbits=1  rst=off  rst_latency=2  en=off  use_dcount=off  use_percent_full_port=off  use_almost_empty=off  almost_empty_thresh=2  use_almost_full=off  use_rd_rst_busy=off  use_wr_rst_busy=off  almost_full_thresh=14  explicit_period=off  dbl_ovrd=off  simulation_type=fast_sim  block_type=fifo
  Logical : xbsIndex_r4/Logical  logical_function=OR  inputs=2  en=off  latency=2  precision=User Defined  arith_type=Boolean  n_bits=1  bin_pt=0  align_bp=on  dbl_ovrd=off  block_type=logical
  Logical1 : xbsIndex_r4/Logical  logical_function=AND  inputs=2  en=off  latency=1  precision=User Defined  arith_type=Boolean  n_bits=1  bin_pt=0  align_bp=on  dbl_ovrd=off  block_type=logical
  Mux1 : xbsIndex_r4/Mux  inputs=2  en=off  latency=1  precision=User Defined  arith_type="Signed  (2's comp)"  n_bits=16  bin_pt=14  quantization=Truncate  overflow=Flag as error  dbl_ovrd=off  block_type=mux
  Mux2 : xbsIndex_r4/Mux  inputs=2  en=off  latency=1  precision=User Defined  arith_type="Signed  (2's comp)"  n_bits=32  bin_pt=14  quantization=Truncate  overflow=Flag as error  dbl_ovrd=off  block_type=mux
  Mux3 : xbsIndex_r4/Mux  inputs=2  en=off  latency=1  precision=Full  arith_type=Unsigned  n_bits=1  bin_pt=0  quantization=Truncate  overflow=Wrap  dbl_ovrd=off  block_type=mux
  Register : xbsIndex_r4/Register  init=0  rst=on  en=on  dbl_ovrd=off  block_type=register
  Register1 : xbsIndex_r4/Register  init=0  rst=on  en=on  dbl_ovrd=off  block_type=register
  Relational1 : xbsIndex_r4/Relational  mode=a=b  op_type=Bool  en=off  latency=1  dbl_ovrd=off  block_type=relational
  Relational2 : xbsIndex_r4/Relational  mode=a=b  op_type=Bool  en=off  latency=1  dbl_ovrd=off  block_type=relational
  Terminator1 : Terminator
  Terminator{6..8,10,12} (5 alike) : Terminator  Commented=on
  Terminator2 : Terminator
  probe{1..5} (5 alike) : xbsIndex_r4/Gateway Out  Commented=on  inherit_from_input=off  hdl_port=on  rows=1  columns=1  UseAsDAC=off  DACChannel='1'  interface=None  automatic_assignment=on  address_offset=hex2dec('00')  intf_name=''  intf_description=''  timing_constraint=None  locs_specified=off  LOCs={}  io_standard={}  block_type=gatewayout
  tvalid_out : Outport
  data_out : Outport  Port=2
  wires:
  Register/1 -> Counter2/2
  Mux2/1 -> AddSub1/2, probe3/1
  Mux1/1 -> AddSub1/1, probe4/1
  Counter2/1 -> probe2/1, Relational1/1
  Constant5/1 -> Mux2/3
  FIFO1/3 -> Terminator1/1
  Constant7/1 -> Register/1
  FIFO1/2 -> Terminator2/1
  probe1/1 -> Terminator6/1  "add_sel_counter"
  probe2/1 -> Terminator7/1  "acc_counter"
  probe5/1 -> Terminator12/1  "Test_rst"
  Constant4/1 -> Delay18/1, FIFO1/2
  Delay19/1 -> Counter3/1
  Delay21/1 -> Counter3/2
  Constant9/1 -> Register1/1
  Relational1/1 -> Logical/1, Register1/3
  Counter3/1 -> probe1/1, Relational2/1
  Register1/1 -> Mux3/3, Delay21/1
  Delay18/1 -> FIFO1/3
  AddSub1/1 -> FIFO1/1
  Constant10/1 -> Relational2/2
  Relational2/1 -> Register1/2, Delay19/1
  rst/1 -> Logical/2, Register/2
  Logical/1 -> Counter2/1, probe5/1
  FIFO1/1 -> Mux2/2, Delay2/1
  probe4/1 -> Terminator10/1  "acc_a"
  data_in/1 -> Mux1/3
  probe3/1 -> Terminator8/1  "acc_b"
  acc_length/1 -> Relational1/2
  tvalid_in/1 -> Mux3/1, Delay3/1, Register/3, Mux1/1
  Constant1/1 -> Mux1/2
  Mux3/1 -> Mux2/1, Logical1/2
  Constant2/1 -> Mux3/2
  Logical1/1 -> tvalid_out/1
  Delay2/1 -> data_out/1
  Delay3/1 -> Logical1/1
